simulink library "Navigation_Lib"  (R2014a)
settings: Solver=ode45  StartTime=0.0  StopTime=10.0  RelTol=1e-3
undefined symbols (not defined in the file or in its folder): DiscIntNeverNeededParam, gyro_x_offset, gyro_y_offset, gyro_z_offset
libraries: simulink x7, aerolibutil x5, vrlib x4, aerolibtransform2 x3, dspmtrx3 x2
(part 3 of 3)

== system Navigation_Lib/Navigation Subsystem/CheckSum Pre-Processing/Magnetometer/CheckSum Correction/Generate Sample Holding Pulse/Transition Logic Detection ==
  Input : Inport
  Constant : Constant  Value=0
  Constant1 : Constant
  Logical Operator : Logic  AllPortsSameDT=off  OutDataTypeStr=boolean
  Relational Operator : RelationalOperator  Operator===  OutDataTypeStr=boolean
  Relational Operator1 : RelationalOperator  Operator===  OutDataTypeStr=boolean
  Unit Delay : UnitDelay  SampleTime=-1
  Transition Detect : Outport
  wires:
  Logical Operator/1 -> Transition Detect/1  "Transition_Detect"
  Constant1/1 -> Relational Operator1/1
  Constant/1 -> Relational Operator/2
  Relational Operator/1 -> Logical Operator/2
  Input/1 -> Unit Delay/1, Relational Operator1/2
  Unit Delay/1 -> Relational Operator/1
  Relational Operator1/1 -> Logical Operator/1

== system Navigation_Lib/Navigation Subsystem/CheckSum Pre-Processing/RateGyro Processing/CheckSum Correction/Generate Sample Holding Pulse/Transition Logic Detection ==
  Input : Inport
  Constant : Constant  Value=0
  Constant1 : Constant
  Logical Operator : Logic  AllPortsSameDT=off  OutDataTypeStr=boolean
  Relational Operator : RelationalOperator  Operator===  OutDataTypeStr=boolean
  Relational Operator1 : RelationalOperator  Operator===  OutDataTypeStr=boolean
  Unit Delay : UnitDelay  SampleTime=-1
  Transition Detect : Outport
  wires:
  Logical Operator/1 -> Transition Detect/1  "Transition_Detect"
  Constant1/1 -> Relational Operator1/1
  Constant/1 -> Relational Operator/2
  Relational Operator/1 -> Logical Operator/2
  Input/1 -> Unit Delay/1, Relational Operator1/2
  Unit Delay/1 -> Relational Operator/1
  Relational Operator1/1 -> Logical Operator/1

== system Navigation_Lib/Navigation Subsystem/CheckSum Pre-Processing/TempFilter/CheckSum Correction/Generate Sample Holding Pulse/Transition Logic Detection ==
  Input : Inport
  Constant : Constant  Value=0
  Constant1 : Constant
  Logical Operator : Logic  AllPortsSameDT=off  OutDataTypeStr=boolean
  Relational Operator : RelationalOperator  Operator===  OutDataTypeStr=boolean
  Relational Operator1 : RelationalOperator  Operator===  OutDataTypeStr=boolean
  Unit Delay : UnitDelay  SampleTime=-1
  Transition Detect : Outport
  wires:
  Logical Operator/1 -> Transition Detect/1  "Transition_Detect"
  Constant1/1 -> Relational Operator1/1
  Constant/1 -> Relational Operator/2
  Relational Operator/1 -> Logical Operator/2
  Input/1 -> Unit Delay/1, Relational Operator1/2
  Unit Delay/1 -> Relational Operator/1
  Relational Operator1/1 -> Logical Operator/1

== system Navigation_Lib/Navigation Subsystem/CheckSum Pre-Processing/Ultrasound Processing/CheckSum Correction/Generate Sample Holding Pulse/Transition Logic Detection ==
  Input : Inport
  Constant : Constant  Value=0
  Constant1 : Constant
  Logical Operator : Logic  AllPortsSameDT=off  OutDataTypeStr=boolean
  Relational Operator : RelationalOperator  Operator===  OutDataTypeStr=boolean
  Relational Operator1 : RelationalOperator  Operator===  OutDataTypeStr=boolean
  Unit Delay : UnitDelay  SampleTime=-1
  Transition Detect : Outport
  wires:
  Logical Operator/1 -> Transition Detect/1  "Transition_Detect"
  Constant1/1 -> Relational Operator1/1
  Constant/1 -> Relational Operator/2
  Relational Operator/1 -> Logical Operator/2
  Input/1 -> Unit Delay/1, Relational Operator1/2
  Unit Delay/1 -> Relational Operator/1
  Relational Operator1/1 -> Logical Operator/1

== matlab function Navigation_Lib/Navigation Subsystem/Attitude Determination/Calculate DCM/Matrix Re-Order ==
  data: M_in input; M_out output
function M_out = MatrixFormat(M_in)
%#codegen

% SL3D coordinate system is different. This EML block is responsible for
% re-ordering the matrix in a format that SL3D can understand

M_out = M_in ; %set size

%re-order diagonal
M_out(1,1) = M_in(2,2);
M_out(2,2) = M_in(3,3);
M_out(3,3) = M_in(1,1);

%re-order bottom half
M_out(2,1) = M_in(3,2) ;
M_out(3,1) = M_in(1,2) ;
M_out(3,2) = M_in(1,3);

%re-order upper half
M_out(1,2) = M_in(2,3);
M_out(1,3) = M_in(2,1) ;
M_out(2,3) = M_in(3,1);

== matlab function Navigation_Lib/Navigation Subsystem/Attitude Determination/Magnetometer Processing/Magnetometer Heading Calculation/Compensate for Magnetic Declination (~60 degrees in Boston)_ ==
  data: vector_in input; y output
function y = fcn(vector_in)
%#codegen

% %  WHY WAS THIS COMMENTED OUT???
% %  Reason: While the intention to rotate 60 degrees up north was in good
% %  intention, the math was not correct: you are rotating in the global
% %  reference frame, an axis which stays fixed. we want to rotate upwards
% %  along an axis which is perpindicular to the XY coordinates
% %

%transform the pitch up, recall that in SL3D the x-axis = z-axis
%                                                y-axis = x-axis

rotation = 1*pi/3;
C_term = cos(rotation);
S_term = sin(rotation);
MatrixY = [C_term 0 -S_term; 0 1 0; S_term 0 C_term ];
MatrixX = [1 0 0; 0 C_term -S_term; 0 S_term C_term ];


y = MatrixY*vector_in;

== matlab function Navigation_Lib/Navigation Subsystem/Attitude Determination/Magnetometer Processing/Magnetometer Heading Calculation/Compensate for Magnetic Declination (~67 degrees in Boston)_2 ==
  data: vector_in input; y output; declination_ang input
function y = fcn(vector_in, declination_ang)

B_xy = norm([vector_in(1) vector_in(2)]);
B_z = vector_in(3);

Declination_Angle = -atan2(B_z,B_xy);


% Declination_Angle = declination_ang*pi/180;

rot_axis = [vector_in(2) -vector_in(1)]; %find a vector perpindicular to the XY vector, such that we can pitch around it
rot_axis = rot_axis/norm(rot_axis);
%rotate by this amount
% for i=1:1:45;
% rot_angle = i*(pi/180) ;

%Define new rotation matrix
C_term = cos(Declination_Angle);
S_term = sin(Declination_Angle);
t = 1-C_term;
ux = rot_axis(1);
uy = rot_axis(2);
uz = 0; 

new_rot = [(t*ux^2 + C_term) (t*ux*uy-S_term*uz) (t*ux*uz+S_term*uy)
           (t*ux*uy+S_term*uz) (t*uy^2+C_term)     (t*uy*uz - S_term*ux)
           (t*ux*uz - S_term*uy) (t*uy*uz+S_term*ux) (t*uz^2 + C_term)];


y = new_rot*vector_in;

== stateflow chart Navigation_Lib/Navigation Subsystem/CheckSum Pre-Processing/Accelerometer Processing/CheckSum Correction/Generate Sample Holding Pulse/Chart ==
  state Begin_State0
    entry: output =0;
  state Begin_State
    entry: output =1;
  state End_State
    entry: output=0;
  (default) -> Begin_State0
  Begin_State0 -> Begin_State : [if_transition==1]
  Begin_State -> End_State [order 1] : after(HoldDataTicks,tick)
  End_State -> Begin_State : [if_transition==1]
  Begin_State -> Begin_State [order 2] : [if_transition==1]
  data: output output; if_transition input; HoldDataTicks input

== stateflow chart Navigation_Lib/Navigation Subsystem/CheckSum Pre-Processing/Magnetometer/CheckSum Correction/Generate Sample Holding Pulse/Chart ==
  state Begin_State0
    entry: output =0;
  state Begin_State
    entry: output =1;
  state End_State
    entry: output=0;
  (default) -> Begin_State0
  Begin_State0 -> Begin_State : [if_transition==1]
  Begin_State -> End_State [order 1] : after(HoldDataTicks,tick)
  End_State -> Begin_State : [if_transition==1]
  Begin_State -> Begin_State [order 2] : [if_transition==1]
  data: output output; if_transition input; HoldDataTicks input

== stateflow chart Navigation_Lib/Navigation Subsystem/CheckSum Pre-Processing/RateGyro Processing/CheckSum Correction/Generate Sample Holding Pulse/Chart ==
  state Begin_State0
    entry: output =0;
  state Begin_State
    entry: output =1;
  state End_State
    entry: output=0;
  (default) -> Begin_State0
  Begin_State0 -> Begin_State : [if_transition==1]
  Begin_State -> End_State [order 1] : after(HoldDataTicks,tick)
  End_State -> Begin_State : [if_transition==1]
  Begin_State -> Begin_State [order 2] : [if_transition==1]
  data: output output; if_transition input; HoldDataTicks input

== stateflow chart Navigation_Lib/Navigation Subsystem/CheckSum Pre-Processing/Ultrasound Processing/CheckSum Correction/Generate Sample Holding Pulse/Chart ==
  state Begin_State0
    entry: output =0;
  state Begin_State
    entry: output =1;
  state End_State
    entry: output=0;
  (default) -> Begin_State0
  Begin_State0 -> Begin_State : [if_transition==1]
  Begin_State -> End_State [order 1] : after(HoldDataTicks,tick)
  End_State -> Begin_State : [if_transition==1]
  Begin_State -> Begin_State [order 2] : [if_transition==1]
  data: output output; if_transition input; HoldDataTicks input

== matlab function Navigation_Lib/Navigation Subsystem/CheckSum Pre-Processing/Ultrasound Processing/Height Calculation ==
  data: u input double; y output double; prev_good_height output double; z_1 input double
function [y,prev_good_height] = fcn(u,z_1)
%#codegen



if u<10000
    
    height = ((u - 880) /26.553);
    prev_good_height = height;
else
    
%     height = u;
%     prev_good_height = height;
    height =  z_1;
    prev_good_height = z_1; 
end

y = height;

== matlab function Navigation_Lib/Navigation Subsystem/LogicCheck ==
  data: u input; y output
function y = fcn(u)
%#codegen

if u > 70 && u < 110
   y = 1;
else
   y = 0;
end

== matlab function Navigation_Lib/Navigation Subsystem/SL3D Visualization/Matrix Re-Order ==
  data: M_in input; M_out output
function M_out = MatrixFormat(M_in)
%#codegen

% SL3D coordinate system is different. This EML block is responsible for
% re-ordering the matrix in a format that SL3D can understand

M_out = M_in ; %set size

%re-order diagonal
M_out(1,1) = M_in(2,2);
M_out(2,2) = M_in(3,3);
M_out(3,3) = M_in(1,1);

%re-order bottom half
M_out(2,1) = M_in(3,2) ;
M_out(3,1) = M_in(1,2) ;
M_out(3,2) = M_in(1,3);

%re-order upper half
M_out(1,2) = M_in(2,3);
M_out(1,3) = M_in(2,1) ;
M_out(2,3) = M_in(3,1);

== matlab function Navigation_Lib/Navigation Subsystem/SL3D Visualization/Subsystem/Compensate 
for Magnetic Declination 
(~60 degrees in Boston)_ ==
  data: vector_in input; y output
function y = fcn(vector_in)
%#codegen

% %  WHY WAS THIS COMMENTED OUT???
% %  Reason: While the intention to rotate 60 degrees up north was in good
% %  intention, the math was not correct: you are rotating in the global
% %  reference frame, an axis which stays fixed. we want to rotate upwards
% %  along an axis which is perpindicular to the XY coordinates
% %

%transform the pitch up, recall that in SL3D the x-axis = z-axis
%                                                y-axis = x-axis

rotation = 1*pi/3;
C_term = cos(rotation);
S_term = sin(rotation);
MatrixY = [C_term 0 -S_term; 0 1 0; S_term 0 C_term ];
MatrixX = [1 0 0; 0 C_term -S_term; 0 S_term C_term ];


y = MatrixY*vector_in;
